simulink model "lr_cont"  (R2015a)
settings: Solver=ode45  StartTime=0.0  StopTime=.04  MaxStep=1e-4  RelTol=1e-3
values from neighbouring files (symbols this model uses):
  k1 = 2*alphac*L - R    (= 637.884901332)    [Sim_lr_cont.m]
  ki = alphac^2*L    (= 604019.789347)    [Sim_lr_cont.m]
  kt = alphac*L    (= 320.442450666)    [Sim_lr_cont.m]
  LAct = .17    (= 0.17)    [Sim_lr_cont.m]
  RAct = 3    [Sim_lr_cont.m]
  umax = 350    [Sim_lr_cont.m]
settings Model: Creator=mhink  LastModifiedBy=mhinkkan
settings DataIOCC: SaveFormat=Dataset
settings HardwareCC: ProdBitPerPointer=64  ProdLargestAtomicFloat=Float  ProdIntDivRoundTo=Zero  ProdEndianess=LittleEndian  ProdHWDeviceType=Specified
settings GRTTargetCC: GeneratePreprocessorConditionals=Use local settings

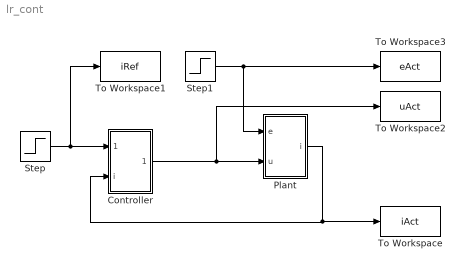
== system lr_cont ==
  Controller : Subsystem
  Plant : Subsystem
  Step : Step  Time=2e-3  After=10  SampleTime=0
  Step1 : Step  Time=20e-3  After=100  SampleTime=0
  To Workspace : ToWorkspace  VariableName=iAct  SaveFormat=Timeseries  SampleTime=-1
  To Workspace1 : ToWorkspace  VariableName=iRef  SaveFormat=Timeseries  SampleTime=-1
  To Workspace2 : ToWorkspace  VariableName=uAct  SaveFormat=Timeseries  SampleTime=-1
  To Workspace3 : ToWorkspace  VariableName=eAct  SaveFormat=Timeseries  SampleTime=-1
  wires:
  Step/1 -> To Workspace1/1, Controller/1(iref)
  Plant/1(i) -> Controller/2(i), To Workspace/1
  Step1/1 -> To Workspace3/1, Plant/1(e)
  Controller/1(uref) -> To Workspace2/1, Plant/2(u)

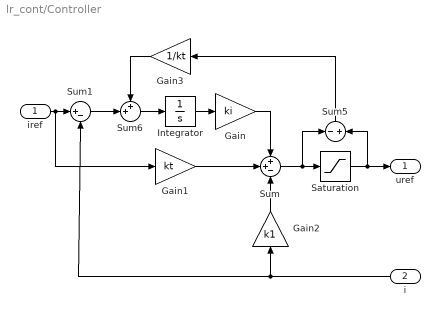
== system lr_cont/Controller ==
  iref : Inport
  i : Inport  Port=2
  Gain : Gain  Gain=ki
  Gain1 : Gain  Gain=kt
  Gain2 : Gain  Gain=k1
  Gain3 : Gain  Gain=1/kt
  Integrator : Integrator
  Saturation : Saturate  UpperLimit=umax  LowerLimit=-umax
  Sum : Sum  Inputs=++-
  Sum1 : Sum  Inputs=|+-
  Sum5 : Sum  Inputs=-|+
  Sum6 : Sum  Inputs=++|
  uref : Outport
  wires:
  Sum6/1 -> Integrator/1
  Gain1/1 -> Sum/2
  Sum/1 -> Sum5/1, Saturation/1
  Integrator/1 -> Gain/1
  iref/1 -> Gain1/1, Sum1/1
  Saturation/1 -> Sum5/2, uref/1
  i/1 -> Gain2/1, Sum1/2
  Sum1/1 -> Sum6/2
  Gain2/1 -> Sum/3
  Gain/1 -> Sum/1
  Gain3/1 -> Sum6/1
  Sum5/1 -> Gain3/1

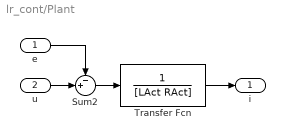
== system lr_cont/Plant ==
  e : Inport
  u : Inport  Port=2
  Sum2 : Sum  Inputs=-+|
  Transfer Fcn : TransferFcn  Denominator=[LAct RAct]
  i : Outport
  wires:
  Sum2/1 -> Transfer Fcn/1
  Transfer Fcn/1 -> i/1
  e/1 -> Sum2/1
  u/1 -> Sum2/2
